simulink model "linear_model"  (R2015b)
settings: Solver=VariableStepAuto  StartTime=0.0  StopTime=10.0  RelTol=1e-3
undefined symbols (not defined in the file): Ad, Bd, Cd, fset, x0
settings Model: Creator=mgreiff  LastModifiedBy=mgreiff

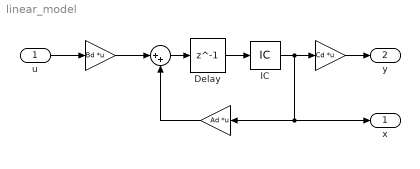
== system linear_model ==
  u : Inport  PortDimensions=1
  " " : Sum  Inputs=|++
  "  " : Gain  Gain=Bd  Multiplication=Matrix(K*u)
  "    " : Gain  Gain=Ad  Multiplication=Matrix(K*u)
  "       " : Gain  Gain=Cd  Multiplication=Matrix(K*u)
  Delay : Delay  DelayLength=1  SampleTime=fset.h
  IC : InitialCondition  Value=x0
  x : Outport
  y : Outport  Port=2
  wires:
  u/1 -> "  "/1
  " "/1 -> Delay/1
  "  "/1 -> " "/1
  Delay/1 -> IC/1
  "    "/1 -> " "/2
  "       "/1 -> y/1
  IC/1 -> x/1, "    "/1, "       "/1
